simulink model "Steer_Request_Saturation"  (R2022a)
settings: Solver=VariableStepAuto  StartTime=0.0  StopTime=10  RelTol=1e-3
libraries: simulink x1
settings Model: Creator=maxju  LastModifiedBy=maxju

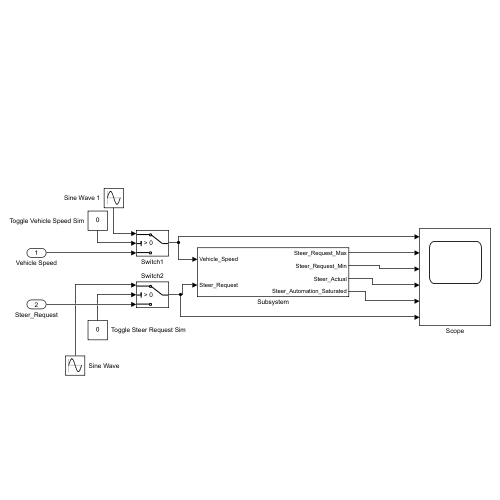
[thumbnail: Simulink's stored preview of the top-level diagram]
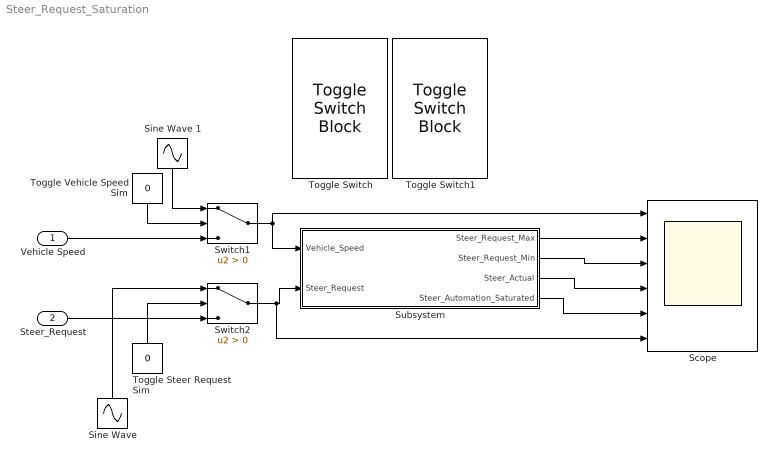
== system Steer_Request_Saturation ==
  Vehicle Speed : Inport
  Steer_Request : Inport  Port=2
  Scope : Scope  NumInputPorts=6
  Sine Wave : Sin  Amplitude=100  SampleTime=0
  Sine Wave 1 : Sin  Amplitude=50  Bias=50  SampleTime=0
  Subsystem : Subsystem
  Switch1 : Switch  Criteria=u2 > Threshold  SaturateOnIntegerOverflow=off  InputSameDT=off
  Switch2 : Switch  Criteria=u2 > Threshold  SaturateOnIntegerOverflow=off  InputSameDT=off
  Toggle Steer Request Sim : Constant  Value=0
  Toggle Switch : ToggleSwitchBlock
      settings: Values={{'Off', 'On'}, [0 1]}
  Toggle Switch1 : ToggleSwitchBlock
      settings: Values={{'Off', 'On'}, [0 1]}
  Toggle Vehicle Speed Sim : Constant  Value=0
  wires:
  Sine Wave 1/1 -> Switch1/1
  Subsystem/1(Steer_Request_Max) -> Scope/2
  Subsystem/2(Steer_Request_Min) -> Scope/3
  Subsystem/3(Steer_Actual) -> Scope/4
  Subsystem/4(Steer_Automation_Saturated) -> Scope/5
  Toggle Vehicle Speed Sim/1 -> Switch1/2
  Switch1/1 -> Scope/1, Subsystem/1(Vehicle_Speed)
  Vehicle Speed/1 -> Switch1/3
  Steer_Request/1 -> Switch2/3
  Toggle Steer Request Sim/1 -> Switch2/2
  Switch2/1 -> Scope/6, Subsystem/2(Steer_Request)
  Sine Wave/1 -> Switch2/1

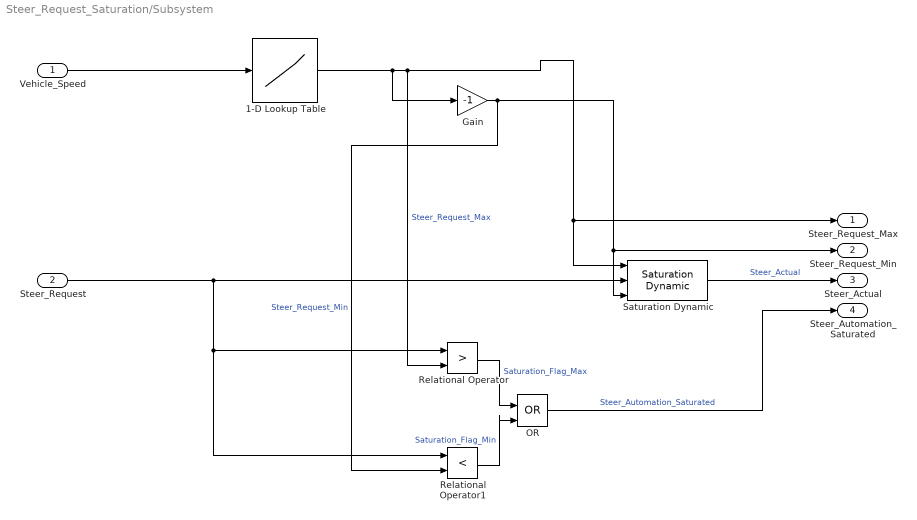
== system Steer_Request_Saturation/Subsystem ==
  Vehicle_Speed : Inport
  Steer_Request : Inport  Port=2
  1-D Lookup Table : Lookup_n-D  NumberOfTableDimensions=1  BreakpointsForDimension1=[0,10,20,30,50]  Table=[100,100,60,40,30]  InternalRulePriority=Speed  RndMeth=Simplest
  Gain : Gain  Gain=-1
  OR : Logic  Operator=OR  IconShape=distinctive  AllPortsSameDT=off  OutDataTypeStr=boolean
  Relational Operator : RelationalOperator  Operator=>  OutDataTypeStr=boolean  RndMeth=Simplest  InputSameDT=off
  Relational Operator1 : RelationalOperator  Operator=<  OutDataTypeStr=boolean  RndMeth=Simplest  InputSameDT=off
  Saturation Dynamic : simulink/Discontinuities/Saturation Dynamic  OutMin=[]  OutMax=[]  OutDataTypeStr=Inherit: Same as second input  OutDataType=fixdt(1, 16)  OutScaling=2^-10  DoSatur=off
  Steer_Request_Max : Outport
  Steer_Request_Min : Outport  Port=2
  Steer_Actual : Outport  Port=3
  Steer_Automation_Saturated : Outport  Port=4
  wires:
  1-D Lookup Table/1 -> Relational Operator/2, Steer_Request_Max/1, Saturation Dynamic/1, Gain/1  "Steer_Request_Max"
  OR/1 -> Steer_Automation_Saturated/1  "Steer_Automation_Saturated"
  Relational Operator1/1 -> OR/2  "Saturation_Flag_Min"
  Relational Operator/1 -> OR/1  "Saturation_Flag_Max"
  Steer_Request/1 -> Saturation Dynamic/2, Relational Operator1/1, Relational Operator/1
  Gain/1 -> Relational Operator1/2, Steer_Request_Min/1, Saturation Dynamic/3  "Steer_Request_Min"
  Vehicle_Speed/1 -> 1-D Lookup Table/1
  Saturation Dynamic/1 -> Steer_Actual/1  "Steer_Actual"
